simulink model "without_sssc"  (Simulink 7.4)
settings: Solver=ode23tb  SolverMode=SingleTasking  StartTime=0  StopTime=10  MaxStep=1/60  RelTol=1e-4  AbsTol=1e-3
undefined symbols (not defined in the file): D1, Delta
libraries: powerlib x22, powerlib_extras x8
Description:
  | Copyright 2008-2009 The MathWorks(TM), Inc.
settings Model: Creator=hyp01  LastModifiedBy=Bharath  ExtModeAutoUpdateStatusClock=off
settings DataIOCC: LimitDataPoints=off  SaveFinalState=on  SaveOutput=off  SaveTime=off  SignalLoggingName=sigsOut
settings OptimizationCC: BooleanDataType=off  InitFltsAndDblsToZero=on
settings DebuggingCC: CheckExecutionContextPreStartOutputMsg=on  CheckExecutionContextRuntimeOutputMsg=on  SignalResolutionControl=TryResolveAllWithWarning  SolverPrmCheckMsg=none  MultiTaskDSMMsg=warning  MultiTaskCondExecSysMsg=none  SigSpecEnsureSampleTimeMsg=none  UnconnectedLineMsg=none  StrictBusMsg=None
settings HardwareCC: TargetUnknown=on
settings RTWCC: IncludeERTFirstTime=on
settings CodeAppCC: IgnoreCustomStorageClasses=off

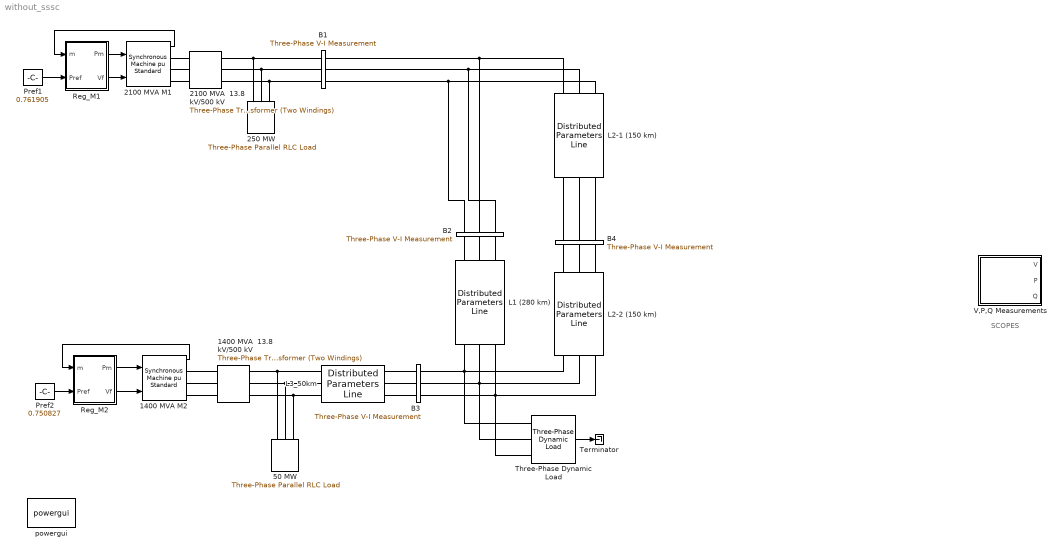
== system without_sssc ==
  note: SCOPES
  1400 MVA M2 : powerlib/Machines/Synchronous Machine pu Standard  DialogController=POWERSYS.PowerSysDialog  SystemSampleTime=-1  PresetModel=No  MechanicalLoad=Mechanical power Pm  ShowDetailedParameters=on  RotorType=Salient-pole  NominalParameters="[1400E6  13800   60 ]"  Reactances1=[ 31 32 33 34 35 36 37 ]  Reactances2=[ 1.305, 0.296, 0.252, 0.474, 0.243, 0.18 ]  dAxisTimeConstants=Short-circuit  qAxisTimeConstants=Open-circuit  TimeConstants1=[]  TimeConstants2=[]  TimeConstants3=[]  TimeConstants4=[]  TimeConstants5=[ 1.01, 0.053, 0.1 ]  TimeConstants6=[]  TimeConstants7=[]  TimeConstants8=[]  StatorResistance=2.8544e-3  Mechanical="[ 3.7 0  32]"  PolePairs=32  InitialConditions=[0 -71.2244 0.745111 0.745111 0.745111 -3.89206 -123.892 116.108 1.33295]  SetSaturation=off  Saturation=[0.6404,0.7127,0.8441,0.9214,0.9956,1.082,1.19,1.316,1.457;0.7,0.7698,0.8872,0.9466,0.9969,1.046,1.1,1.151,1.201]  Units=per unit standard parameters  LoadFlowParameters=[2 1000000000 13938 0 0]  TsPowergui=0  TsBlock=-1  IterativeModel=Forward Euler
      settings: AttributesFormatString=\n\n
  1400 MVA  13.8 kV/500 kV : powerlib/Elements/Three-Phase Transformer (Two Windings)  DialogController=POWERSYS.PowerSysDialog  SystemSampleTime=-1  Winding1Connection=Delta (D1)  UNITS=pu  NominalPower=[ 1400e6 60 ]  Winding1="[ 13.8e3 0.002  0.0]"  Winding2Connection=Yg  Winding2=[ 500e3 0.002 0.12]  SetSaturation=off  Rm=500  Lm=500  Saturation="[ 0,0  ;  0.005,1.2  ;  1.0,1.4 ]"  Hysteresis=off  DataFile='basic_model'  SetInitialFlux=off  InitialFluxes=[ 0.8 , -0.8 , 0.7 ]  Measurements=None  MoreParameters=off  BreakLoop=off  DataType=off  TransfoNumber=0
  2100 MVA M1 : powerlib/Machines/Synchronous Machine pu Standard  DialogController=POWERSYS.PowerSysDialog  SystemSampleTime=-1  PresetModel=No  MechanicalLoad=Mechanical power Pm  ShowDetailedParameters=on  RotorType=Salient-pole  NominalParameters="[2100E6  13800   60 ]"  Reactances1=[ 31 32 33 34 35 36 37 ]  Reactances2=[ 1.305, 0.296, 0.252, 0.474, 0.243, 0.18 ]  dAxisTimeConstants=Short-circuit  qAxisTimeConstants=Open-circuit  TimeConstants1=[]  TimeConstants2=[]  TimeConstants3=[]  TimeConstants4=[]  TimeConstants5=[ 1.01, 0.053, 0.1 ]  TimeConstants6=[]  TimeConstants7=[]  TimeConstants8=[]  StatorResistance=2.8544e-3  Mechanical="[ 3.7 0  32]"  PolePairs=32  InitialConditions=[0 -58.9841 0.763417 0.763417 0.763417 14.3746 -105.625 134.375 1.2256]  SetSaturation=off  Saturation=[0.6404,0.7127,0.8441,0.9214,0.9956,1.082,1.19,1.316,1.457;0.7,0.7698,0.8872,0.9466,0.9969,1.046,1.1,1.151,1.201]  Units=per unit standard parameters  LoadFlowParameters=[1 1600000000 0 0 0]  TsPowergui=0  TsBlock=-1  IterativeModel=Forward Euler
      settings: AttributesFormatString=\n\n
  2100 MVA  13.8 kV/500 kV : powerlib/Elements/Three-Phase Transformer (Two Windings)  DialogController=POWERSYS.PowerSysDialog  SystemSampleTime=-1  Winding1Connection=Delta (D1)  UNITS=pu  NominalPower=[ 2100e6 60 ]  Winding1="[ 13.8e3 0.002  0.0]"  Winding2Connection=Yg  Winding2=[ 500e3 0.002 0.12]  SetSaturation=off  Rm=500  Lm=500  Saturation="[ 0,0  ;  0.005,1.2  ;  1.0,1.4 ]"  Hysteresis=off  DataFile='basic_model'  SetInitialFlux=off  InitialFluxes=[ 0.8 , -0.8 , 0.7 ]  Measurements=None  MoreParameters=off  BreakLoop=off  DataType=off  TransfoNumber=0
  250 MW : powerlib/Elements/Three-Phase Parallel RLC Load  DialogController=POWERSYS.PowerSysDialog  PhysicalDomain=powersysdomain  SubClassName=unknown  LeftPortType=p1  RightPortType=p1  LConnTagsString=A|B|C  Configuration=Y (grounded)  NominalVoltage=500e3  NominalFrequency=60  ActivePower=250e6  InductivePower=0  CapacitivePower=0  Measurements=None
  50 MW : powerlib/Elements/Three-Phase Parallel RLC Load  DialogController=POWERSYS.PowerSysDialog  PhysicalDomain=powersysdomain  SubClassName=unknown  LeftPortType=p1  RightPortType=p1  LConnTagsString=A|B|C  Configuration=Y (grounded)  NominalVoltage=500e3  NominalFrequency=60  ActivePower=50e6  InductivePower=0  CapacitivePower=0  Measurements=None
  B1 : powerlib/Measurements/Three-Phase V-I Measurement  DialogController=POWERSYS.PowerSysDialog  SystemSampleTime=-1  VoltageMeasurement=phase-to-ground  SetLabelV=on  LabelV=Vabc_B1  Vpu=on  CurrentMeasurement=yes  SetLabelI=on  LabelI=Iabc_B1  Ipu=on  Pbase=100e6  Vbase=500e3  OutputType=Complex  PhasorSimulation=on  PSBequivalent=0
  B2 : powerlib/Measurements/Three-Phase V-I Measurement  DialogController=POWERSYS.PowerSysDialog  SystemSampleTime=-1  VoltageMeasurement=phase-to-ground  SetLabelV=on  LabelV=Vabc_B2  Vpu=on  CurrentMeasurement=yes  SetLabelI=on  LabelI=Iabc_B2  Ipu=on  Pbase=100e6  Vbase=500e3  OutputType=Complex  PhasorSimulation=on  PSBequivalent=0
  B3 : powerlib/Measurements/Three-Phase V-I Measurement  DialogController=POWERSYS.PowerSysDialog  SystemSampleTime=-1  VoltageMeasurement=phase-to-ground  SetLabelV=on  LabelV=Vabc_B3  Vpu=on  CurrentMeasurement=yes  SetLabelI=on  LabelI=Iabc_B3  Ipu=on  Pbase=100e6  Vbase=500e3  OutputType=Complex  PhasorSimulation=on  PSBequivalent=0
  B4 : powerlib/Measurements/Three-Phase V-I Measurement  DialogController=POWERSYS.PowerSysDialog  SystemSampleTime=-1  VoltageMeasurement=phase-to-ground  SetLabelV=on  LabelV=Vabc_B4  Vpu=on  CurrentMeasurement=yes  SetLabelI=on  LabelI=Iabc_B4  Ipu=on  Pbase=100e6  Vbase=500e3  OutputType=Complex  PhasorSimulation=on  PSBequivalent=0
  L1 (280 km) : powerlib/Elements/Distributed Parameters Line  DialogController=POWERSYS.PowerSysDialog  SystemSampleTime=-1  Phases=3  Frequency=60  Resistance=[0.01273*2 0.3864]  Inductance="[0.9337e-3  4.1264e-3]"  Capacitance=[12.74e-9 7.751e-9]  Length=280  x1=[0 8.89645577442958e-009 334295.859601952 -388307.040483474;0.000316703277517616 9.74697269381243e-009 349496.470628607 -401814.971295117;0.000633406555035232 1.04587114498752e-008 359720.923436262 -409601.828963071;0.000950109832552847 1.10215382502669e-008 364823.641462206 -411556.743595817;0.00126681311007046 1.14274395227657e-008 364731.971806115 -407651.880965159;0.00158351638758808 1.16706360131502e-008 359447.219667759 -397942.838812153]  x2=[0 1.58135150877377e-008 326957.267092308 -300762.807240537;0.000316703277517616 1.45762964920414e-008 351600.818975475 -326624.337352209;0.000633406555035232 1.31315394412042e-008 371238.250762479 -347835.364476204;0.000950109832552847 1.14998144996728e-008 385589.963156047 -364093.884341159;0.00126681311007046 9.70435429541733e-009 394451.615347084 -375168.406863327;0.00158351638758808 7.7707227319479e-009 397697.034435174 -380901.252120587]  x3=[0 4.78762731382045e-011 303.049528810583 -248.45417874666;0.000316703277517616 4.98285079561003e-011 389.090038582176 -238.824176092287;0.000633406555035232 5.10712805612295e-011 469.590653802218 -225.79377604729;0.000950109832552847 5.15868962595593e-011 543.405200383911 -209.548506471692;0.00126681311007046 5.13680136742496e-011 609.48270101125 -190.319668790576;0.00158351638758808 5.04177492727543e-011 666.882339036655 -168.38104470622]  x4=[0 -1.66695486741975e-011 1840.28703947018 -1997.16244392116;0.000316703277517616 -1.79688508524766e-011 1953.15698949011 -2206.1962819777;0.000633406555035232 -1.90123111199785e-011 2038.21773677684 -2383.81812396588;0.000950109832552847 -1.97850726073991e-011 2094.25817972478 -2527.49897613852;0.00126681311007046 -2.02761326759419e-011 2120.4804101025 -2635.19309922915;0.00158351638758808 -2.04784995737542e-011 2116.51107373283 -2705.36713584854]  x5=0.00158351638758808  Measurements=None
      settings: AttributesFormatString=\n
  L2-1 (150 km) : powerlib/Elements/Distributed Parameters Line  DialogController=POWERSYS.PowerSysDialog  SystemSampleTime=-1  Phases=3  Frequency=60  Resistance=[0.01273*2 0.3864]  Inductance="[0.9337e-3  4.1264e-3]"  Capacitance=[12.74e-9 7.751e-9]  Length=150  x1=[0 1.06631957472729e-008 528575.008044035 -104008.340677356;0.000169662470098723 1.09576180597628e-008 534185.226898297 -106520.245493019;0.000339324940197445 1.12072275906221e-008 537610.817141422 -108596.520185923;0.000508987410296168 1.14110035251685e-008 538837.769321111 -110228.673527053;0.000678649880394891 1.15681124919149e-008 537861.06563698 -111410.030586613;0.000848312350493614 1.16779119707644e-008 534684.70046159 -112135.760032133]  x2=[0 1.12102566466695e-008 452877.865316144 -224109.767951009;0.000169662470098723 1.08994562718456e-008 460881.940992254 -230961.335480664;0.000339324940197445 1.05440809765291e-008 467001.172565703 -236868.35285028;0.000508987410296168 1.01455841199646e-008 471210.534544019 -241806.662448409;0.000678649880394891 9.7055954133281e-009 473492.812125765 -245756.068335712;0.000848312350493614 9.22591425478458e-009 473838.671602982 -248700.418839203]  x3=[0 5.03366752110245e-011 1132.4777522743 823.600259236226;0.000169662470098723 5.03870476405904e-011 1078.66515964024 658.838544734247;0.000339324940197445 5.02313548696162e-011 1020.44120807873 491.382413647024;0.000508987410296168 4.98702336264592e-011 958.044012955066 321.916702313459;0.000678649880394891 4.9305160769258e-011 891.728756724428 151.134465544774;0.000848312350493614 4.85384472461052e-011 821.766645325921 -20.265857724497]  x4=[0 -2.24155842536306e-011 2366.9284833825 -1966.50401303967;0.000169662470098723 -2.21085784497538e-011 2493.1887524405 -1843.60532337669;0.000339324940197445 -2.17111563808797e-011 2609.25276146118 -1713.16694011253;0.000508987410296168 -2.12249433626827e-011 2714.64584970505 -1575.72231009243;0.000678649880394891 -2.06519278344104e-011 2808.93699672377 -1431.83353323244;0.000848312350493614 -1.99944532268706e-011 2891.74058508131 -1282.08906372956]  x5=0.000848312350493614  Measurements=None
      settings: AttributesFormatString=\n
  L2-2 (150 km) : powerlib/Elements/Distributed Parameters Line  DialogController=POWERSYS.PowerSysDialog  SystemSampleTime=-1  Phases=3  Frequency=60  Resistance=[0.01273*2 0.3864]  Inductance="[0.9337e-3  4.1264e-3]"  Capacitance=[12.74e-9 7.751e-9]  Length=150  x1=[0 1.12102566466695e-008 452877.865316144 -224109.767951009;0.000169662470098723 1.08994562718456e-008 460881.940992254 -230961.335480664;0.000339324940197445 1.05440809765291e-008 467001.172565703 -236868.35285028;0.000508987410296168 1.01455841199646e-008 471210.534544019 -241806.662448409;0.000678649880394891 9.7055954133281e-009 473492.812125765 -245756.068335712;0.000848312350493614 9.22591425478458e-009 473838.671602982 -248700.418839203]  x2=[0 1.26263811164877e-008 360390.287842327 -336025.973612996;0.000169662470098723 1.17435113979424e-008 370404.799394193 -346917.602015504;0.000339324940197445 1.08126148720214e-008 378904.486346438 -356390.460147126;0.000508987410296168 9.83749857621318e-009 385854.587986175 -364405.807369106;0.000678649880394891 8.82215039122221e-009 391226.68085628 -370930.863746717;0.000848312350493614 7.7707227319479e-009 394998.794997281 -375938.944107602]  x3=[0 5.21329558890495e-011 943.619635074684 328.256203996976;0.000169662470098723 5.15997239759913e-011 875.869352259969 155.272390438735;0.000339324940197445 5.08554674451629e-011 804.537073631413 -18.3464322691257;0.000508987410296168 4.99032300424961e-011 729.914522974967 -191.890224559016;0.000678649880394891 4.8746906082116e-011 652.306880125247 -364.649253711216;0.000848312350493614 4.73912245199733e-011 572.031532887973 -535.916996409627]  x4=[0 -1.76113950117055e-011 1918.29602622305 -2269.45294683733;0.000169662470098723 -1.83969316317323e-011 2070.78047500476 -2174.38207731416;0.000339324940197445 -1.91072313092603e-011 2214.79616417783 -2070.41875427777;0.000508987410296168 -1.97393891698756e-011 2349.75412051881 -1957.98815094257;0.000678649880394891 -2.02908199115525e-011 2475.10241372734 -1837.55006870412;0.000848312350493614 -2.07592683776252e-011 2590.32841362589 -1709.59705671406]  x5=0.000848312350493614  Measurements=None
      settings: AttributesFormatString=\n
  L3_50km : powerlib/Elements/Distributed Parameters Line  DialogController=POWERSYS.PowerSysDialog  SystemSampleTime=-1  Phases=3  Frequency=60  Resistance=[0.01273*2 0.3864]  Inductance="[0.9337e-3  4.1264e-3]"  Capacitance=[12.74e-9 7.751e-9]  Length=50  x1=[0 9.5033175587461e-009 379157.487669875 -356677.001923957;5.65541566995743e-005 9.16481687605871e-009 381630.870577428 -359496.443471433;0.000113108313399149 8.82215039122221e-009 383930.785894486 -362152.478474395;0.000169662470098723 8.47547386084344e-009 386056.188210944 -364643.899651076;0.000226216626798297 8.12494486426684e-009 388006.111440337 -366969.574543748;0.000282770783497871 7.7707227319479e-009 389779.669258967 -369128.446033476]  x2=[0 6.17508952887797e-009 403956.898634192 -329350.162630786;5.65541566995743e-005 5.7015204552018e-009 405876.280837106 -331684.576697347;0.000113108313399149 5.22535979606498e-009 407611.174871205 -333868.225905087;0.000169662470098723 4.74682398689922e-009 409160.79215278 -335900.117691833;0.000226216626798297 4.26613054274375e-009 410524.428314346 -337779.328475664;0.000282770783497871 3.78349795937538e-009 411701.463524811 -339505.00407472]  x3=[0 8.07097434751968e-011 2933.87682999196 -2485.42955924302;5.65541566995743e-005 7.8953571378657e-011 2971.19813941196 -2461.57404813521;0.000113108313399149 7.71615114993304e-011 3007.16891190776 -2436.59964609934;0.000169662470098723 7.53343784052543e-011 3041.77279722127 -2410.51770507175;0.000226216626798297 7.3473002606746e-011 3074.99406640319 -2383.34008041271;0.000282770783497871 7.15782301788995e-011 3106.81761896257 -2355.07912551769]  x4=[0 -5.6752304518297e-011 -77.0352665948822 -9.89362387375485;5.65541566995743e-005 -5.60486173903004e-011 -96.1809881188012 -54.4791076131124;0.000113108313399149 -5.53194537629983e-011 -115.282991260517 -99.03982826264;0.000169662470098723 -5.45651450725169e-011 -134.332593340734 -143.555531064566;0.000226216626798297 -5.37860341844921e-011 -153.321135498685 -188.00598172366;0.000282770783497871 -5.29824752382215e-011 -172.239986627955 -232.370975604587]  x5=0.000282770783497871  Measurements=None
      settings: AttributesFormatString=\n
  Pref1 : Constant  Value=0.761905  OutDataType=sfix(16)  OutScaling=2^0
  Pref2 : Constant  Value=0.750827  OutDataType=sfix(16)  OutScaling=2^0
  Reg_M1 : Subsystem
  Reg_M2 : Subsystem
  Terminator : Terminator
  Three-Phase Dynamic Load : powerlib/Elements/Three-Phase Dynamic Load  DialogController=POWERSYS.PowerSysDialog  SystemSampleTime=-1  NominalVoltage=[ 500e3 60 ]  ActiveReactivePowers=[2.2e+009 1e+008]  PositiveSequence=[1.00208 20.9514]  ExternalControl=off  NpNq=[1.3 2]  TimeConstants="[0  0  0  0]"  MinimumVoltage=0.7  LoadFlowParameters=[4 2200000000 0 0 100000000]
  V,P,Q Measurements : Subsystem
      mask Display: disp('V P Q\nMeasurements')
  powergui : powerlib/powergui  Priority=2  SystemSampleTime=-1  SimulationMode=Phasor  SampleTime=0  frequency=60  SPID=off  DisableSnubberDevices=off  DisableRonSwitches=off  DisableVfSwitches=off  SwTol=0  Interpol=off  frequencyindice=60  echomessages=on  HookPort=off  DisplayEquations=off  FunctionMessages=off  EnableUseOfTLC=off  x0status=blocks  RestoreLinks=warning  Frange=[0:2:500]  Ylog=off  Xlog=on  ShowGrid=off  save=off  variable=ZData  ZoomFFT=on  StartTime=0.0  cycles=1  DisplayStyle=1  fundamental=60  FreqAxis=off  MaxFrequency=1000  frequencyindicesteady=1  RmsSteady=1  display=off  Ts=0  methode=off
  wires:
  Reg_M1/1(Pm) -> 2100 MVA M1/1
  Reg_M1/2(Vf) -> 2100 MVA M1/2
  Pref1/1 -> Reg_M1/2(Pref)
  2100 MVA M1/1 -> Reg_M1/1(m)
  Reg_M2/1(Pm) -> 1400 MVA M2/1
  Reg_M2/2(Vf) -> 1400 MVA M2/2
  Pref2/1 -> Reg_M2/2(Pref)
  1400 MVA M2/1 -> Reg_M2/1(m)
  Three-Phase Dynamic Load/1 -> Terminator/1
  connections:
  2100 MVA M1/RConn1 -- 2100 MVA  13.8 kV/500 kV/LConn1
  2100 MVA M1/RConn2 -- 2100 MVA  13.8 kV/500 kV/LConn2
  2100 MVA M1/RConn3 -- 2100 MVA  13.8 kV/500 kV/LConn3
  250 MW/LConn1 -- 2100 MVA  13.8 kV/500 kV/RConn1 -- B1/LConn1
  250 MW/LConn2 -- 2100 MVA  13.8 kV/500 kV/RConn2 -- B1/LConn2
  250 MW/LConn3 -- 2100 MVA  13.8 kV/500 kV/RConn3 -- B1/LConn3
  L2-1 (150 km)/LConn1 -- B1/RConn1 -- B2/LConn3
  L2-1 (150 km)/LConn2 -- B1/RConn2 -- B2/LConn2
  L2-1 (150 km)/LConn3 -- B1/RConn3 -- B2/LConn1
  1400 MVA M2/RConn1 -- 1400 MVA  13.8 kV/500 kV/LConn1
  1400 MVA M2/RConn2 -- 1400 MVA  13.8 kV/500 kV/LConn2
  1400 MVA M2/RConn3 -- 1400 MVA  13.8 kV/500 kV/LConn3
  B3/RConn1 -- L2-2 (150 km)/RConn1 -- L1 (280 km)/RConn1 -- Three-Phase Dynamic Load/LConn1
  B3/RConn2 -- L2-2 (150 km)/RConn2 -- L1 (280 km)/RConn2 -- Three-Phase Dynamic Load/LConn2
  B3/RConn3 -- L1 (280 km)/RConn3 -- L2-2 (150 km)/RConn3 -- Three-Phase Dynamic Load/LConn3
  B4/RConn1 -- L2-2 (150 km)/LConn1
  B4/RConn2 -- L2-2 (150 km)/LConn2
  B4/RConn3 -- L2-2 (150 km)/LConn3
  L2-1 (150 km)/RConn1 -- B4/LConn1
  L2-1 (150 km)/RConn2 -- B4/LConn2
  L2-1 (150 km)/RConn3 -- B4/LConn3
  1400 MVA  13.8 kV/500 kV/RConn1 -- 50 MW/LConn1 -- L3_50km/RConn1
  1400 MVA  13.8 kV/500 kV/RConn2 -- 50 MW/LConn2 -- L3_50km/RConn2
  1400 MVA  13.8 kV/500 kV/RConn3 -- 50 MW/LConn3 -- L3_50km/RConn3
  B2/RConn1 -- L1 (280 km)/LConn1
  B2/RConn2 -- L1 (280 km)/LConn2
  B2/RConn3 -- L1 (280 km)/LConn3
  L3_50km/LConn1 -- B3/LConn1
  L3_50km/LConn2 -- B3/LConn2
  L3_50km/LConn3 -- B3/LConn3

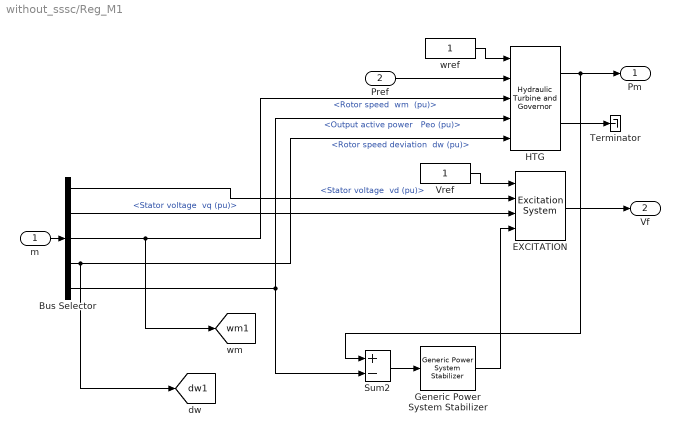
== system without_sssc/Reg_M1 ==
  m : Inport  OutDataType=sfix(16)  OutScaling=2^0
  Pref : Inport  Port=2  OutDataType=sfix(16)  OutScaling=2^0
  Bus Selector : BusSelector  OutputSignals="dq0 components.Stator voltage  vd (pu),dq0 components.Stator voltage  vq (pu),Mechanical.Rotor speed  wm  (pu),Mechanical.Rotor speed deviation  dw (pu),Output active power   Peo (pu)"
  EXCITATION : powerlib/Machines/Excitation System  DialogController=POWERSYS.PowerSysDialog  SystemSampleTime=-1  tr=20e-3  reg=[ 200, 0.001 ]  exc=[ 1, 0 ]  tgr=[ 0, 0 ]  damp=[ 0.001, 0.1 ]  sat=[ 0, 0 ]  lim="[ 0,  7, 0 ]"  v0=[1,1.2256]
  Generic Power System Stabilizer : powerlib/Machines/Generic Power System Stabilizer  DialogController=POWERSYS.PowerSysDialog  SystemSampleTime=-1  Tsensor=15e-3  K=2.5/10  Twashout=1  Tleadlag1="[0.06  1]"  Tleadlag2="[0  0]"  VSlimits=[-0.15 0.15]  Vinit=0  Plot_On=off  MagdB_On=on  FreqRange=logspace(-2,2,500)
  HTG : powerlib/Machines/Hydraulic Turbine and Governor  DialogController=POWERSYS.PowerSysDialog  SystemSampleTime=-1  sm="[ 10/3  0.07 ]"  gate="[  0.01  0.97518  -0.1  0.1 ]"  reg="[  0.05  1.163  0.105  0  0.01  ]"  hyd="[  0  2.67  ]"  dref=0  po=0.763568
  Sum2 : Sum  Inputs=+-  OutDataType=sfix(16)  OutScaling=2^0  SaturateOnIntegerOverflow=on  InputSameDT=on  OutDataTypeStr=Inherit: Same as first input
  Terminator : Terminator
  Vref : Constant  OutDataType=sfix(16)  OutScaling=2^0
  wref : Constant  OutDataType=sfix(16)  OutScaling=2^0
  Pm : Outport  OutDataType=sfix(16)  OutScaling=2^0  InitialOutput=0
  Vf : Outport  Port=2  OutDataType=sfix(16)  OutScaling=2^0  InitialOutput=0
  tag scope: dw1=global, wm1=global
  wires:
  Sum2/1 -> Generic Power System Stabilizer/1
  Bus Selector/1 -> EXCITATION/2  "<Stator voltage  vd (pu)>"
  EXCITATION/1 -> Vf/1
  Bus Selector/2 -> EXCITATION/3  "<Stator voltage  vq (pu)>"
  HTG/1 -> Sum2/1, Pm/1
  wref/1 -> HTG/1
  Pref/1 -> HTG/2
  Bus Selector/3 -> [wm1], HTG/3  "<Rotor speed  wm  (pu)>"
  Bus Selector/5 -> Sum2/2, HTG/4  "<Output active power   Peo (pu)>"
  Bus Selector/4 -> [dw1], HTG/5  "<Rotor speed deviation  dw (pu)>"
  m/1 -> Bus Selector/1
  Vref/1 -> EXCITATION/1
  HTG/2 -> Terminator/1
  Generic Power System Stabilizer/1 -> EXCITATION/4

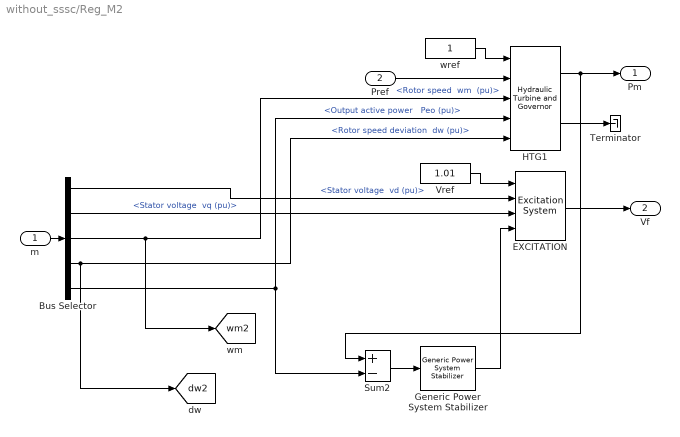
== system without_sssc/Reg_M2 ==
  m : Inport  OutDataType=sfix(16)  OutScaling=2^0
  Pref : Inport  Port=2  OutDataType=sfix(16)  OutScaling=2^0
  Bus Selector : BusSelector  OutputSignals="dq0 components.Stator voltage  vd (pu),dq0 components.Stator voltage  vq (pu),Mechanical.Rotor speed  wm  (pu),Mechanical.Rotor speed deviation  dw (pu),Output active power   Peo (pu)"
  EXCITATION : powerlib/Machines/Excitation System  DialogController=POWERSYS.PowerSysDialog  SystemSampleTime=-1  tr=20e-3  reg=[ 200, 0.001 ]  exc=[ 1, 0 ]  tgr=[ 0, 0 ]  damp=[ 0.001, 0.1 ]  sat=[ 0, 0 ]  lim="[ 0,  7, 0 ]"  v0=[1.01,1.33295]
  Generic Power System Stabilizer : powerlib/Machines/Generic Power System Stabilizer  DialogController=POWERSYS.PowerSysDialog  SystemSampleTime=-1  Tsensor=15e-3  K=2.5/10  Twashout=1  Tleadlag1="[0.06  1]"  Tleadlag2="[0  0]"  VSlimits=[-0.15 0.15]  Vinit=0  Plot_On=off  MagdB_On=on  FreqRange=logspace(-2,2,500)
  HTG1 : powerlib/Machines/Hydraulic Turbine and Governor  DialogController=POWERSYS.PowerSysDialog  SystemSampleTime=-1  sm="[ 10/3  0.07 ]"  gate="[  0.01  0.97518  -0.1  0.1 ]"  reg="[  0.05  1.163  0.105  0  0.01  ]"  hyd="[  0  2.67  ]"  dref=0  po=0.752412
  Sum2 : Sum  Inputs=+-  OutDataType=sfix(16)  OutScaling=2^0  SaturateOnIntegerOverflow=on  InputSameDT=on  OutDataTypeStr=Inherit: Same as first input
  Terminator : Terminator
  Vref : Constant  Value=1.01  OutDataType=sfix(16)  OutScaling=2^0
  wref : Constant  OutDataType=sfix(16)  OutScaling=2^0
  Pm : Outport  OutDataType=sfix(16)  OutScaling=2^0  InitialOutput=0
  Vf : Outport  Port=2  OutDataType=sfix(16)  OutScaling=2^0  InitialOutput=0
  tag scope: dw2=global, wm2=global
  wires:
  HTG1/2 -> Terminator/1
  Vref/1 -> EXCITATION/1
  m/1 -> Bus Selector/1
  Bus Selector/4 -> [dw2], HTG1/5  "<Rotor speed deviation  dw (pu)>"
  Bus Selector/5 -> Sum2/2, HTG1/4  "<Output active power   Peo (pu)>"
  Bus Selector/3 -> [wm2], HTG1/3  "<Rotor speed  wm  (pu)>"
  Pref/1 -> HTG1/2
  wref/1 -> HTG1/1
  HTG1/1 -> Pm/1, Sum2/1
  Bus Selector/2 -> EXCITATION/3  "<Stator voltage  vq (pu)>"
  EXCITATION/1 -> Vf/1
  Bus Selector/1 -> EXCITATION/2  "<Stator voltage  vd (pu)>"
  Sum2/1 -> Generic Power System Stabilizer/1
  Generic Power System Stabilizer/1 -> EXCITATION/4

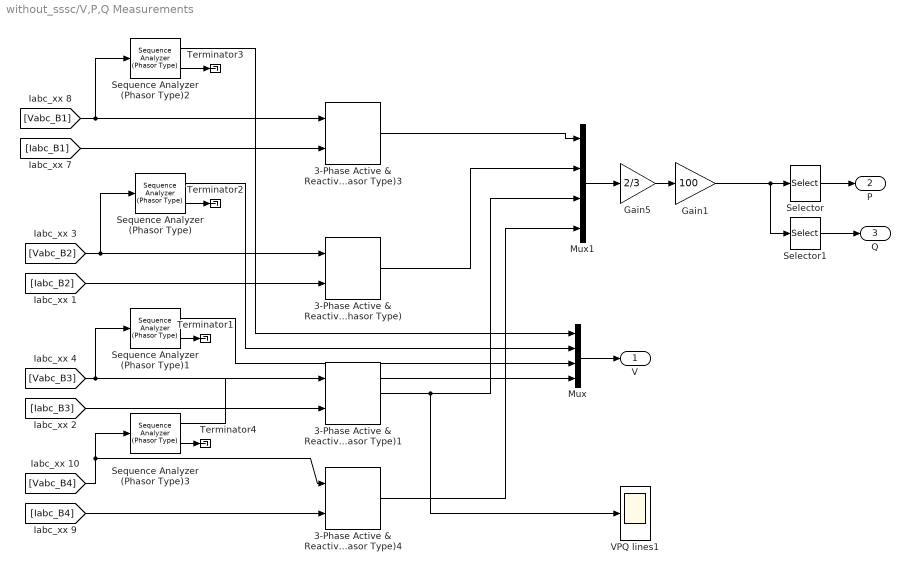
== system without_sssc/V,P,Q Measurements ==
  3-Phase Active & Reactive Power (Phasor Type){,1,3..4} (4 alike) : powerlib_extras/Phasor Library/3-Phase Active & Reactive Power (Phasor Type)  DialogController=POWERSYS.PowerSysDialog  SystemSampleTime=-1
  Gain1 : Gain  Gain=100  ParameterDataType=sfix(16)  ParameterScaling=2^0  OutDataType=sfix(16)  OutScaling=2^0  SaturateOnIntegerOverflow=on  OutDataTypeStr=Inherit: Same as input  ParamDataTypeStr=Inherit: Same as input
  Gain5 : Gain  Gain=2/3  ParameterDataType=sfix(16)  ParameterScaling=2^0  OutDataType=sfix(16)  OutScaling=2^0  SaturateOnIntegerOverflow=on  OutDataTypeStr=Inherit: Same as input  ParamDataTypeStr=Inherit: Same as input
  Mux : Mux
  Mux1 : Mux
  Selector : Selector  InputPortWidth=8  IndexOptions=Index vector (dialog)  Indices=[1 3 5 7 ]  OutputSizes=1
  Selector1 : Selector  InputPortWidth=8  IndexOptions=Index vector (dialog)  Indices=[1 3 5 7 ]+1  OutputSizes=1
  Sequence Analyzer (Phasor Type){,1..3} (4 alike) : powerlib_extras/Phasor Library/Sequence Analyzer (Phasor Type)  DialogController=POWERSYS.PowerSysDialog  SystemSampleTime=-1  seq=Positive
  Terminator{1..4} (4 alike) : Terminator
  VPQ lines1 : Scope
      settings: YMin=7.5  YMax=12
  V : Outport  OutDataType=sfix(16)  OutScaling=2^0
  P : Outport  Port=2  OutDataType=sfix(16)  OutScaling=2^0
  Q : Outport  Port=3  OutDataType=sfix(16)  OutScaling=2^0
  wires:
  [Iabc_B1] -> 3-Phase Active & Reactive Power (Phasor Type)3/2
  [Vabc_B1] -> 3-Phase Active & Reactive Power (Phasor Type)3/1, Sequence Analyzer (Phasor Type)2/1
  Sequence Analyzer (Phasor Type)2/1 -> Mux/1
  Sequence Analyzer (Phasor Type)2/2 -> Terminator3/1
  3-Phase Active & Reactive Power (Phasor Type)3/1 -> Mux1/1
  Sequence Analyzer (Phasor Type)3/1 -> Mux/4
  3-Phase Active & Reactive Power (Phasor Type)4/1 -> Mux1/4
  Sequence Analyzer (Phasor Type)3/2 -> Terminator4/1
  [Iabc_B4] -> 3-Phase Active & Reactive Power (Phasor Type)4/2
  [Vabc_B4] -> 3-Phase Active & Reactive Power (Phasor Type)4/1, Sequence Analyzer (Phasor Type)3/1
  Selector1/1 -> Q/1
  Selector/1 -> P/1
  Mux1/1 -> Gain5/1
  Mux/1 -> V/1
  3-Phase Active & Reactive Power (Phasor Type)1/1 -> Mux1/3, VPQ lines1/1
  3-Phase Active & Reactive Power (Phasor Type)/1 -> Mux1/2
  Sequence Analyzer (Phasor Type)1/1 -> Mux/3
  Sequence Analyzer (Phasor Type)/1 -> Mux/2
  Sequence Analyzer (Phasor Type)1/2 -> Terminator1/1
  [Iabc_B3] -> 3-Phase Active & Reactive Power (Phasor Type)1/2
  [Vabc_B3] -> Sequence Analyzer (Phasor Type)1/1, 3-Phase Active & Reactive Power (Phasor Type)1/1
  [Iabc_B2] -> 3-Phase Active & Reactive Power (Phasor Type)/2
  [Vabc_B2] -> Sequence Analyzer (Phasor Type)/1, 3-Phase Active & Reactive Power (Phasor Type)/1
  Sequence Analyzer (Phasor Type)/2 -> Terminator2/1
  Gain5/1 -> Gain1/1
  Gain1/1 -> Selector1/1, Selector/1
